simulink model "testBCIRobot"  (Simulink 7.4)
settings: Solver=FixedStepDiscrete  SolverMode=SingleTasking  StartTime=0.0  StopTime=inf  FixedStep=0.002  MaxStep=0.02  RelTol=1e-3  AbsTol=1e-6
CloseFcn:
  | rtwprivate ssgencode ModelCloseRequest MC_AD
settings Model: Creator=fwornle  LastModifiedBy=fw  ExtModeTrigDuration=5000  Value=Nmax  OutDataType=sfix(16)  OutScaling=2^0
settings ConfigSet: Description=rtmc9s12target_R2009b
settings DataIOCC: LimitDataPoints=off  SaveOutput=off  SaveTime=off  SignalLoggingName=sigsOut
settings OptimizationCC: BlockReduction=off  BooleanDataType=off  InitFltsAndDblsToZero=on  OptimizeModelRefInitCode=on  LifeSpan=1
settings DebuggingCC: SaveWithParameterizedLinksMsg=none  SignalResolutionControl=TryResolveAllWithWarning  SolverPrmCheckMsg=none  MultiTaskDSMMsg=warning  MultiTaskCondExecSysMsg=none  StrictBusMsg=None
settings HardwareCC: ProdBitPerInt=16  ProdEndianess=BigEndian  ProdWordSize=16  ProdHWDeviceType=Motorola HC12
settings RTWCC: SystemTargetFile=mc9s12.tlc  GenerateMakefile=off  TemplateMakefile=mc9s12.tmf  ProcessScript=mc9s12_make_rtw_hook  IncludeERTFirstTime=on
settings CodeAppCC: IgnoreCustomStorageClasses=off
settings STFCustomTargetCC: TargetFcnLib=ansi_tfl_tmw.mat  ModelReferenceCompliant=off  IncludeMdlTerminateFcn=off  ERTCustomFileBanners=on  SupportNonInlinedSFcns=off  CPPClassGenCompliant=on  SystemTargetFile=mc9s12.tlc
settings ERTTargetCC: TargetFcnLib=ansi_tfl_tmw.mat  MultiwordLength=2048  ModelReferenceCompliant=off  ParMdlRefBuildCompliant=off  CompOptLevelCompliant=off  IncludeMdlTerminateFcn=off  CombineOutputUpdateFcns=off  ERTFirstTimeCompliant=off  SupportContinuousTime=on  ModelStepFunctionPrototypeControlCompliant=off  ExtModeMexFile=ext_serial_mc9s12_comm  ExtModeMexArgs=1,2,115200  InlinedParameterPlacement=NonHierarchical  ERTCustomFileTemplate=mc9s12_file_process.tlc  GRTInterface=on  ConvertIfToSwitch=off
settings CustomProperty: DataType=RTWOptions_EnumType_C__Users_fw__SVN_rtmc9s12-target_trunk_rtmc9s12_CW_R2009b_bin_mc9s12_1mc9s12_TargetBoard  Value=MiniDragonPlus-RevE
settings EnumStrPairs: String=Dragon12

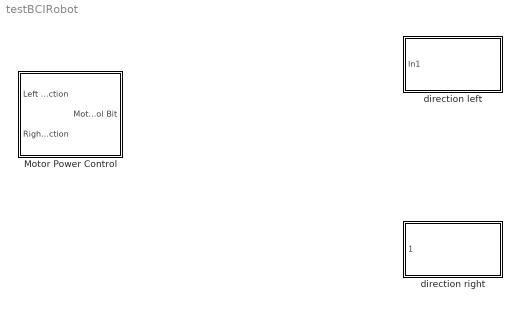
== system testBCIRobot ==
  Motor Power Control : Subsystem
  direction left : Subsystem  Tag=mcTarget_digOut  mask{port=Port A, pin=5, sampletime=0.002, Von=0.5, Voff=0.5}
      mask prompts: port "Port (see hardware manuals for valid options)"; pin "Pin (see hardware manuals for valid options)"; sampletime "Sample time"; Von "On-threshold (Von)"; Voff "Off-threshold (Voff)"
      mask init:
      | [portstr, pinstr, pins] = mbc_digitaloutput(port, pin, sampletime, Von, Voff);
      mask Help: web('digOut_sfcn_9S12.html');
      mask StyleString: popup(Port A|Port B|Port H|Port J|Port M|Port P|Port S|Port T),edit,edit,edit,edit
      mask Display: fprintf('%s\nPins: %s', portstr, pinstr)
  direction right : Subsystem  Tag=mcTarget_digOut  mask{port=Port A, pin=7, sampletime=0.002, Von=0.5, Voff=0.5}
      mask prompts: port "Port (see hardware manuals for valid options)"; pin "Pin (see hardware manuals for valid options)"; sampletime "Sample time"; Von "On-threshold (Von)"; Voff "Off-threshold (Voff)"
      mask init:
      | [portstr, pinstr, pins] = mbc_digitaloutput(port, pin, sampletime, Von, Voff);
      mask Help: web('digOut_sfcn_9S12.html');
      mask StyleString: popup(Port A|Port B|Port H|Port J|Port M|Port P|Port S|Port T),edit,edit,edit,edit
      mask Display: fprintf('%s\nPins: %s', portstr, pinstr)

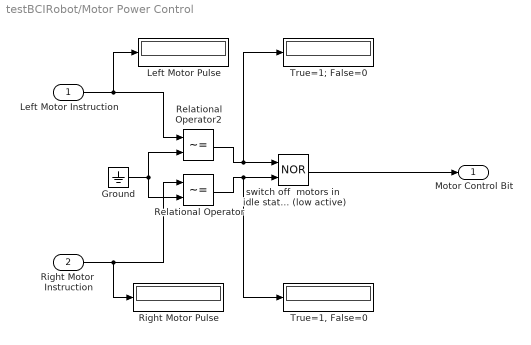
== system testBCIRobot/Motor Power Control ==
  Left Motor Instruction : Inport  OutDataType=sfix(16)  OutScaling=2^0
  Right Motor  Instruction : Inport  Port=2  OutDataType=sfix(16)  OutScaling=2^0
  Ground : Ground
  Left Motor Pulse : Display
  Relational Operator : RelationalOperator  Operator=~=
  Relational Operator2 : RelationalOperator  Operator=~=
  Right Motor Pulse : Display
  "True=1, False=0" : Display
  True=1; False=0 : Display
  switch off  motors in  idle state (low active) : Logic  Operator=NOR  AllPortsSameDT=off
  Motor Control Bit : Outport  OutDataType=sfix(16)  OutScaling=2^0
  wires:
  Right Motor  Instruction/1 -> Relational Operator/1, Right Motor Pulse/1
  Left Motor Instruction/1 -> Relational Operator2/1, Left Motor Pulse/1
  Ground/1 -> Relational Operator2/2, Relational Operator/2
  Relational Operator2/1 -> switch off  motors in  idle state (low active)/1, True=1; False=0/1
  Relational Operator/1 -> switch off  motors in  idle state (low active)/2, "True=1, False=0"/1
  switch off  motors in  idle state (low active)/1 -> Motor Control Bit/1

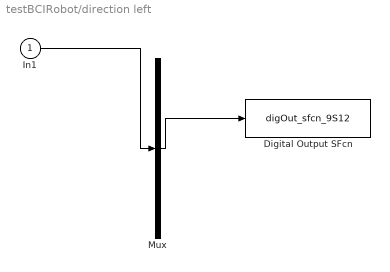
== system testBCIRobot/direction left ==
  In1 : Inport  OutDataType=sfix(16)  OutScaling=2^0
  Digital Output SFcn : S-Function  Tag=mcTarget_digOut  FunctionName=digOut_sfcn_9S12  Parameters=sampletime, port, pins, Von, Voff  EnableBusSupport=off
  Mux : Mux  Inputs=1
  wires:
  In1/1 -> Mux/1
  Mux/1 -> Digital Output SFcn/1

== system testBCIRobot/direction right ==
